simulink model "latchHigh_th"  (R2018b)
settings: Solver=FixedStepAuto  StartTime=0.0  StopTime=10.0  FixedStep=0.1  RelTol=1e-3
libraries: simulink x2, latchHigh_ul x1
settings Model: Creator=mcobb  LastModifiedBy=mcobb

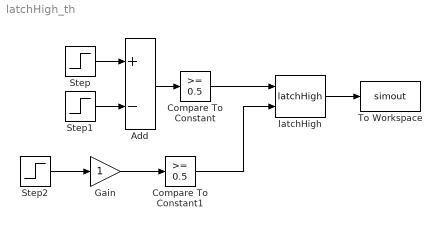
== system latchHigh_th ==
  Add : Sum  Inputs=+-
  Compare To Constant : simulink/Logic and Bit Operations/Compare To Constant  relop=>=  const=0.5  OutDataTypeStr=boolean
  Compare To Constant1 : simulink/Logic and Bit Operations/Compare To Constant  relop=>=  const=0.5  OutDataTypeStr=boolean
  Gain : Gain
  Step : Step  Time=3  SampleTime=0
  Step1 : Step  Time=7  SampleTime=0
  Step2 : Step  Time=4  SampleTime=0
  To Workspace : ToWorkspace  VariableName=simout  SaveFormat=Timeseries  SampleTime=-1
  latchHigh : latchHigh_ul/latchHigh  SystemSampleTime=-1
  wires:
  latchHigh/1 -> To Workspace/1
  Compare To Constant/1 -> latchHigh/1
  Add/1 -> Compare To Constant/1
  Step/1 -> Add/1
  Step1/1 -> Add/2
  Step2/1 -> Gain/1
  Compare To Constant1/1 -> latchHigh/2
  Gain/1 -> Compare To Constant1/1
